simulink model "mavlinkMST_ArucoCamera"  (R2025b)
settings: Solver=ode1  StartTime=0.0  StopTime=inf  FixedStep=0.01  RelTol=1e-3
PreLoadFcn:
  | modelFile = get_param(bdroot,'FileName');                   if ~isempty(modelFile), addpath(fileparts(modelFile)); end; aruco_camera_config;
InitFcn:
  | aruco_camera_config;                       set_param([bdroot '/ArUco Landing Camera'],'MarkerFile',markerImageFile);             set_param([bdroot '/RGB Frames to Python'],'Host',cameraFrameHost);
undefined symbols (not defined in the file or in its folder): uav
libraries: instrumentlib x2, uavmavlinklib x1
settings Model: Creator=y3353li  LastModifiedBy=yangli
settings DebuggingCC: UnderspecifiedInitializationDetection=Classic  MergeDetectMultiDrivingBlocksExec=none
settings ModelReferenceCC: PropagateSignalLabelsOutOfModel=off

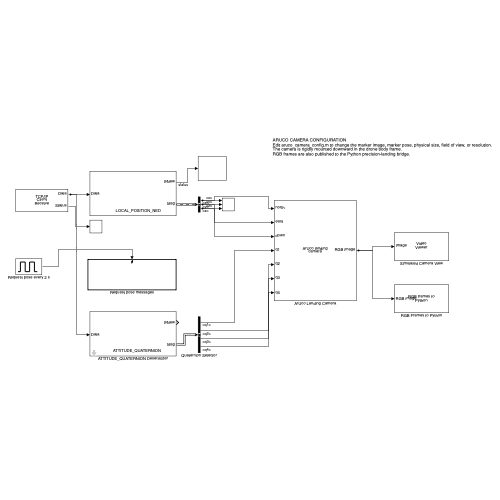
[thumbnail: Simulink's stored preview of the top-level diagram]
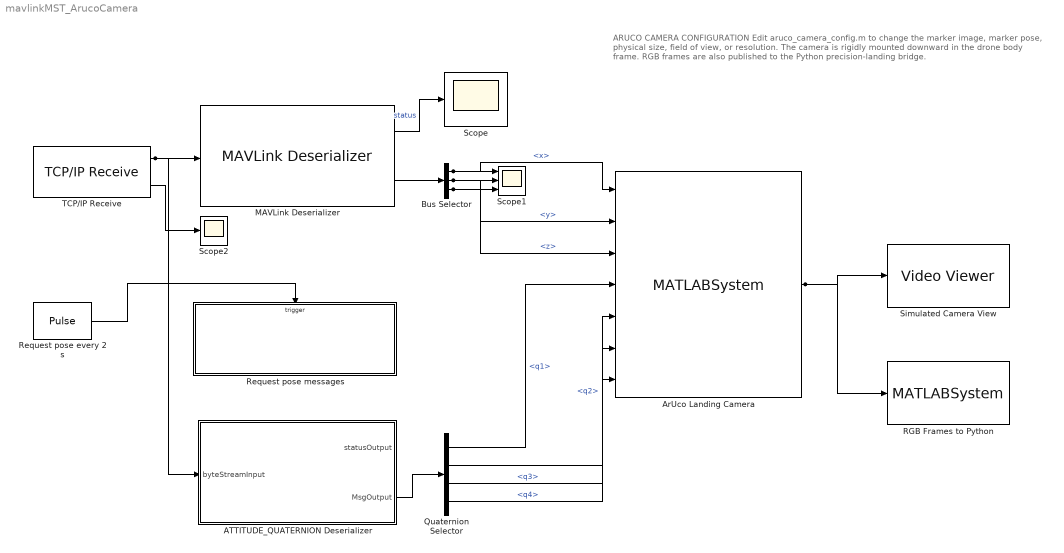
== system mavlinkMST_ArucoCamera ==
  note: ARUCO CAMERA CONFIGURATION
      | Edit aruco_camera_config.m to change the marker image, marker pose, physical size, field of view, or resolution.
      | The camera is rigidly mounted downward in the drone body frame.
      | RGB frames are also published to the Python precision-landing bridge.
  ATTITUDE_QUATERNION Deserializer : Subsystem  InitFcn=uav.sluav.internal.mavlink.util.errorIfBlocksConflict(bdroot(gcb))  mask(MAVLink Deserializer){dialectSource=Select from standard MAVLink dialects, dialect=common.xml, dialectCustom=common.xml, version=2, messageType=ATTITUDE_QUATERNION, inputDataLength=off, SystemIDFilter=off, systemID=1, ComponentIDFilter=off, componentID=1, queueMsg=off, queueMsgSize=50, dropNum=off}
      mask prompts: dialectSource "uav:robotsluav:mavlink:DialectSourcePrompt"; dialect "uav:robotsluav:mavlink:DialectPrompt"; dialectCustom "uav:robotsluav:mavlink:DialectPromptCustom"; version "uav:robotsluav:mavlink:VersionPrompt"; messageType "uav:robotsluav:mavlink:MessageTypePrompt"; inputDataLength "uav:robotsluav:mavlink:InputDataLengthPrompt"; SystemIDFilter "uav:robotsluav:mavlink:FilterbySystemIDPrompt"; systemID "uav:robotsluav:mavlink:SystemIDPrompt"; ComponentIDFilter "uav:robotsluav:mavlink:FilterbyComponentIDPrompt"; componentID "uav:robotsluav:mavlink:ComponentIDPrompt"; queueMsg "uav:robotsluav:mavlink:QueueMessagesPrompt"; queueMsgSize "uav:robotsluav:mavlink:QueueMessagesSizePrompt"; dropNum "uav:robotsluav:mavlink:MsgDroppedPrompt"
      mask help: uav:robotsluav:mavlink:DeserializerDescription
      mask init:
      | uav.sluav.internal.mavlink.block.DeserializerBlockMask.dispatch('maskInitialize', gcb)
      settings: ModelCloseFcn=uav.sluav.internal.mavlink.block.DeserializerBlockMask.dispatch('modelCloseFcn', gcb);
      mask Help: eval("helpview('uav','uavMAVLinkDeserializer')");
      mask TypeOptions dialectSource: uav:robotsluav:mavlink:DialectSourceFromStandard | uav:robotsluav:mavlink:DialectSourceSpecifyOwn
      mask Callback dialectSource: uav.sluav.internal.mavlink.block.DeserializerBlockMask.dispatch('dialectSourceSelect', gcb);
      mask TypeOptions dialect: uav:robotsluav:mavlink:DialectCommon | uav:robotsluav:mavlink:DialectArdupilotmega | uav:robotsluav:mavlink:DialectASLUAV | uav:robotsluav:mavlink:DialectAutoquad | uav:robotsluav:mavlink:DialectIcarous | uav:robotsluav:mavlink:DialectMatrixpilot | uav:robotsluav:mavlink:DialectMinimal | uav:robotsluav:mavlink:DialectPaparazzi | uav:robotsluav:mavlink:DialectSlugs | uav:robotsluav:mavlink:DialectStandard | uav:robotsluav:mavlink:DialectUalberta | uav:robotsluav:mavlink:DialectUAvionix
      mask Callback dialect: uav.sluav.internal.mavlink.block.DeserializerBlockMask.dispatch('dialectEdit', gcb);
      mask Callback dialectCustom: uav.sluav.internal.mavlink.block.DeserializerBlockMask.dispatch('dialectEdit', gcb);
      mask TypeOptions version: 2 | 1
      mask Callback version: uav.sluav.internal.mavlink.block.DeserializerBlockMask.dispatch('versionEdit', gcb);
      mask Callback messageType: uav.sluav.internal.mavlink.block.DeserializerBlockMask.dispatch('messageTypeEdit', gcb);
      mask Callback SystemIDFilter: uav.sluav.internal.mavlink.block.DeserializerBlockMask.dispatch('setSystemIDFilter', gcb);
      mask Callback systemID: uav.sluav.internal.mavlink.block.DeserializerBlockMask.dispatch('setSystemIDFilter', gcb);
      mask Callback ComponentIDFilter: uav.sluav.internal.mavlink.block.DeserializerBlockMask.dispatch('setComponentIDFilter', gcb);
      mask Callback componentID: uav.sluav.internal.mavlink.block.DeserializerBlockMask.dispatch('setComponentIDFilter', gcb);
      mask Callback queueMsg: uav.sluav.internal.mavlink.block.DeserializerBlockMask.dispatch('setQueueMsgSize', gcb);
      mask Callback queueMsgSize: uav.sluav.internal.mavlink.block.DeserializerBlockMask.dispatch('setQueueMsgSize', gcb);
      mask DialogControl MainContainer Prompt: uav:robotsluav:mavlink:MainTabTitle
      mask DialogControl dialectSource Prompt: MAVLink dialect source:
      mask DialogControl dialect Prompt: MAVLink dialect:
      mask DialogControl dialectCustom Prompt: MAVLink dialect:
      mask DialogControl dialectBrowseButton Prompt: uav:robotsluav:mavlink:DialectBrowsePrompt
      mask DialogControl dialectBrowseButton Callback: uav.sluav.internal.mavlink.block.DeserializerBlockMask.dispatch('dialectBrowse', gcb);
      mask DialogControl version Prompt: MAVLink version:
      mask DialogControl messageType Prompt: MAVLink message type:
      mask DialogControl msgSelectButton Prompt: uav:robotsluav:mavlink:MessageSelectPrompt
      mask DialogControl msgSelectButton Callback: uav.sluav.internal.mavlink.block.DeserializerBlockMask.dispatch('messageTypeSelect', gcb, 'uav.sluav.internal.mavlink.dlg.MessageTypeSelector');
      mask DialogControl AdvancedContainer Prompt: uav:robotsluav:mavlink:AdvancedTabTitle
      mask DialogControl inputDataLength Prompt: Input data stream length is available
      mask DialogControl SystemIDFilter Prompt: Filter output MAVLink messages by System ID
      mask DialogControl systemID Prompt: System ID:
      mask DialogControl ComponentIDFilter Prompt: Filter output MAVLink messages by Component ID
      mask DialogControl componentID Prompt: Component ID:
      mask DialogControl queueMsg Prompt: Queue MAVLink messages in output
      mask DialogControl queueMsgSize Prompt: Number of messages to be queued
      mask DialogControl dropNum Prompt: Output number of messages dropped due to checksum mismatch
      mask Display:
      | color('black');
      | text(0.83, 0.10, 'ATTITUDE_QUATERNION', 'horizontalAlignment', 'right');
      | port_label('output', 1, 'IsNew');
      | port_label('output', 2, 'Msg');
      | port_label('input', 1, 'Data');
  ArUco Landing Camera : MATLABSystem  System=ArucoLandingCamera  MarkerFile=/Users/yangli/Desktop/APSM/markers/aruco_6x6_250_id_0.png  MarkerSizeMeters=markerSizeMeters  MarkerNorthMeters=markerNorthMeters  MarkerEastMeters=markerEastMeters  MarkerYawDegrees=markerYawDegrees  GroundDownMeters=groundDownMeters  HorizontalFovDegrees=cameraHorizontalFovDegrees  ImageWidth=cameraImageWidth  ImageHeight=cameraImageHeight  FramePeriodSeconds=cameraFramePeriodSeconds
      mask Type: ArucoLandingCamera
  Bus Selector : BusSelector  OutputSignals=Payload.x,Payload.y,Payload.z
  MAVLink Deserializer : uavmavlinklib/MAVLink Deserializer  dialectSource=Select from standard MAVLink dialects  dialect=common.xml  dialectCustom=common.xml  version=2  messageType=LOCAL_POSITION_NED  inputDataLength=off  SystemIDFilter=off  systemID=1  ComponentIDFilter=off  componentID=1  queueMsg=off  queueMsgSize=50  dropNum=off
  Quaternion Selector : BusSelector  OutputSignals=Payload.q1,Payload.q2,Payload.q3,Payload.q4
  RGB Frames to Python : MATLABSystem  System=ArucoFrameServer  Host=127.0.0.1  Port=cameraFramePort
      mask Type: ArucoFrameServer
  Request pose every 2 s : DiscretePulseGenerator  PulseType=Time based  PhaseDelay=0.1  SampleTime=0.01
  Request pose messages : Subsystem  TreatAsAtomicUnit=on
  Scope : Scope
      settings: ActiveDisplayYMinimum=-1  ActiveDisplayYMaximum=1
  Scope1 : Scope  NumInputPorts=3
      settings: ActiveDisplayYMinimum=-75.175605297088623  ActiveDisplayYMaximum=89.282588481903076
  Scope2 : Scope
      settings: ActiveDisplayYMinimum=-1  ActiveDisplayYMaximum=1  DataLoggingVariableName=ScopeData2
  Simulated Camera View : VideoViewer  FigPos=[2041 741 418 304]
  TCP/IP Receive : instrumentlib/TCP//IP Receive  Host=127.0.0.1  Port=5762  DataSize=256  DataType=uint8  ASCIIFormatting=%f  Terminator=LF  CustomTerminator=10  ByteOrder=big-endian  EnableBlockingMode=off  Timeout=10  SampleTime=0.02  SimulateUsing=Interpreted execution
  wires:
  MAVLink Deserializer/1 -> Scope/1  "status"
  MAVLink Deserializer/2 -> Bus Selector/1
  TCP/IP Receive/1 -> MAVLink Deserializer/1, ATTITUDE_QUATERNION Deserializer/1(byteStreamInput)
  TCP/IP Receive/2 -> Scope2/1
  Request pose every 2 s/1 -> Request pose messages/Trigger
  Bus Selector/1 -> Scope1/1, ArUco Landing Camera/1  "<x>"
  Bus Selector/2 -> Scope1/2, ArUco Landing Camera/2  "<y>"
  Bus Selector/3 -> Scope1/3, ArUco Landing Camera/3  "<z>"
  ATTITUDE_QUATERNION Deserializer/2(MsgOutput) -> Quaternion Selector/1
  Quaternion Selector/1 -> ArUco Landing Camera/4  "<q1>"
  Quaternion Selector/2 -> ArUco Landing Camera/5  "<q2>"
  Quaternion Selector/3 -> ArUco Landing Camera/6  "<q3>"
  Quaternion Selector/4 -> ArUco Landing Camera/7  "<q4>"
  ArUco Landing Camera/1 -> Simulated Camera View/1, RGB Frames to Python/1

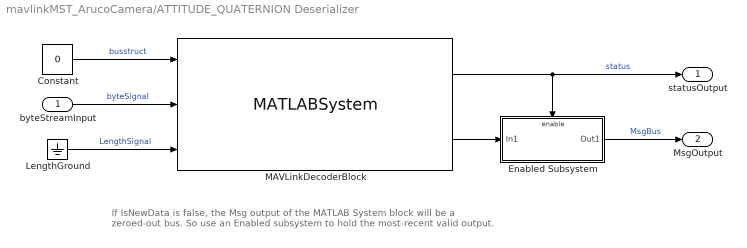
== system mavlinkMST_ArucoCamera/ATTITUDE_QUATERNION Deserializer ==
  note: If IsNewData is false, the Msg output of the MATLAB System block will be a zeroed-out bus. So use an Enabled subsystem to hold the most-recent valid output.
  byteStreamInput : Inport
  Constant : Constant  Value=0  OutDataTypeStr=Bus: SL_Bus_MAVLink_ATTITUDE_QUATERNION_Packet
  Enabled Subsystem : Subsystem  TreatAsAtomicUnit=on
  LengthGround : Ground
  MAVLinkDecoderBlock : MATLABSystem  InitFcn=uav.sluav.internal.mavlink.block.DeserializerBlockMask.dispatch('sysobjInitFcn', gcb);  System=uav.sluav.internal.system.MAVLinkDecoder  MAVLinkMsg=ATTITUDE_QUATERNION  MAVLinkMsgID=31  MAVLinkDialectVersion=2  SLBusName=SL_Bus_MAVLink_ATTITUDE_QUATERNION_Packet  MessageCount=215  MessageDefinitionID="[0      1      2      4      5      6      7      8     11     19     20     21     22     23     24     25     26     27     28     29     30     31     32     33     34     35     36     37     38     39     40     41     42     43     44     45     46     47     48     49     50     51     52     54     55     61     62     63     64     65     66     67     69     70     73     74     75     76     77     80     81     82     83     84     85     86     87     89     90     91     92     93    100    101    102    103    104    105    106    107    108    109    110    111    112    113    114    115    116    117    118    119    120    121    122    123    124    125    126    127    128    129    130    131    132    133    134    135    136    137    138    139    140    141    142    143    144    146    147    148    149    162    230    231    232    233    234    235    241    242    243    244    245    246    247    248    249    250    251    252    253    254    256    257    258    259    260    261    262    263    264    265    266    267    268    269    270    271    275    276    280    281    282    283    284    285    286    287    290    291    299    300    301    310    311    320    321    322    323    324    325    326    327    328    329    330    331    332    333    334    335    336    339    340    350    360    370    371    373    375    380    385    390    395    400    401   9000   9005  12900  12901  12902  12903  12904  12905  12915]"  MessageDefinitionCRC="[50  124  137  237  217  104  119  117   89  137  214  159  220  168   24   23  170  144   67  115   39  246  185  104  237  244  222  212    9  254  230   28   28  132  221  232   11  153   41   39   78  196  132   15    3  167  183  119  191  118  148   21  243  124   38   20  158  152  143   14  106   49   22  143  140    5  150  231  183   63   54   47  175  102  158  208   56   93  138  108   32  185   84   34  174  124  237    4   76  128   56  116  134  237  203  250   87  203  220   25  226   46   29  223   85    6  229  203    1  195  109  168  181   47   72  131  127  103  154  178  200  189  163  105  151   35  150  179   90  104   85   95  130  184   81    8  204   49  170   44   83   46   71  131  187   92  146  179   12  133   49   26  193   35   14  109   59   22  126   18  166    0  123  247   99  137  210   74  221   10   19  217  243   28   95  243   88  243   78  132  228   24  178  160  121   23   91  236  231   72  225  245  199   99  232   11   98  161  117  251  232  147  156  163  110  183  113  117  114  254   49  249  203   49   62]"  MessageDefinitionMinLength="[9   31   12   14   28    3   32   36    6   24   20    2   25   23   30  101   22   26   16   14   28   32   28   28   22   22   21    6    6   37    4    4    2    2    4    2    2    3   13   12   37    4    7   27   25   72   26  181  225   42    6    4   11   18   37   20   35   33    3    4   22   39   37   53   51   53   51   28   56   42   33   81   26   32   32   20   32   62   44   64   84    9  254   16   12   36   44   64   22    6   14   12   97    2    2  113   35    6   79   35   35   22   13  255   14   18   43    8   22   14   36   43   41   32  243   14   93  100   36   60   30    8   42   40   63  182   40   42   32   52   53    6    2   38   19  254   36   30   18   18   51    9   42    9   32  235    5   27   18  255   28   16  255  255    4  213   19   52   31   49   33    9   35   98   32   40   53   23   42   57   96   22   58   17  116   20    2  149  147  146  149  147  146    6    6  158  230  239  109   10   24   84    5   70   20   25   73   50   42  140   20  133  238  156  254    6  137   34   44   59   53   46   46   43  254]"  MessageDefinitionMaxLength="[9   31   12   14   28    3   32   36    6   24   20    2   25   23   52  101   24   29   16   16   28   48   28   28   22   22   37    7    7   38    5    4    2    3    5    3    2    4   21   20   37    5    7   27   25   72   26  181  225   42    6    4   11   38   38   20   35   33   10    4   22   39   37   53   51   53   51   28   56   42   33   81   34  117  117   57  116   63   44   64   84    9  254   16   12   37   44   64   24    6   14   12   97    2    2  113   37    6   79   35   35   24   13  255   39   18   43    8   22   16  120   43   41   32  243   16   93  100   49   78   60    9   42   40   65  182   40   42   32   60   61    6    2   38   19  254   36   30   18   18   54    9   42    9  232  235   13   27   22  255   28   20  255  255    4  213   19   52   31   49   33    9   35   98   32   40   53   23   42   57   98   22   58   17  116   21    3  149  147  146  149  147  146    6    6  167  232  239  109   10   24   84    5   70  252   25   73   50   42  140   20  133  238  156  254    6  137   34   44   59   53   46   46   43  254]"  FilteredSystemID=1  FilteredComponentID=1  OutputMsgQueueSize=50  IsLengthAvailable=off  FilterBySystemID=off  FilterByComponentID=off  QueueOutputMsg=off
      mask Type: uav.sluav.internal.system.MAVLinkDecoder
  statusOutput : Outport  VectorParamsAs1DForOutWhenUnconnected=off
  MsgOutput : Outport  Port=2  VectorParamsAs1DForOutWhenUnconnected=off  LockScale=on
  wires:
  LengthGround/1 -> MAVLinkDecoderBlock/3  "LengthSignal"
  Constant/1 -> MAVLinkDecoderBlock/1  "busstruct"
  MAVLinkDecoderBlock/1 -> Enabled Subsystem/Enable, statusOutput/1  "status"
  Enabled Subsystem/1(Out1) -> MsgOutput/1  "MsgBus"
  MAVLinkDecoderBlock/2 -> Enabled Subsystem/1(In1)
  byteStreamInput/1 -> MAVLinkDecoderBlock/2  "byteSignal"

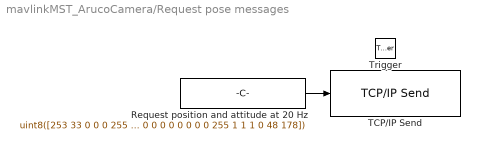
== system mavlinkMST_ArucoCamera/Request pose messages ==
  Trigger : TriggerPort  VariantControl=(inherit)
  Request position and attitude at 20 Hz : Constant  Value=uint8([253 33 0 0 0 255 190 76 0 0 0 0 0 66 0 80 67 71 0 0 0 0 0 0 0 0 0 0 0 0 0 0 0 0 0 0 0 0 255 1 1 1 0 74 217 253 33 0 0 1 255 190 76 0 0 0 0 248 65 0 80 67 71 0 0 0 0 0 0 0 0 0 0 0 0 0 0 0 0 0 0 0 0 255 1 1 1 0 48 178])
  TCP/IP Send : instrumentlib/TCP//IP Send  Host=127.0.0.1  Port=5762  ByteOrder=big-endian  EnableBlockingMode=on  Timeout=2  TransferDelay=off  SimulateUsing=Interpreted execution
  wires:
  Request position and attitude at 20 Hz/1 -> TCP/IP Send/1

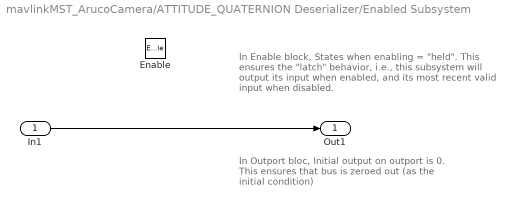
== system mavlinkMST_ArucoCamera/ATTITUDE_QUATERNION Deserializer/Enabled Subsystem ==
  note: In Enable block, States when enabling = "held".
      | This ensures the "latch" behavior, i.e., this subsystem
      | will output its input when enabled, and its most recent
      | valid input when disabled.
  note: In Outport bloc, Initial output on outport is 0.
      | This ensures that bus is zeroed out
      | (as the initial condition)
  In1 : Inport
  Enable : EnablePort
  Out1 : Outport  InitialOutput=0  VectorParamsAs1DForOutWhenUnconnected=off
  wires:
  In1/1 -> Out1/1
